simulink model "rah"  (Simulink 3.00)
settings: Solver=ode15s  SolverMode=SingleTasking  StartTime=0.0  StopTime=60  MaxStep=5  RelTol=1e-6  AbsTol=1e-6
undefined symbols (not defined in the file): Aail, Arud, Bail, Brud, Cail, Crud, Dail, dar, drr, Drud, Ki_2, Kphi, Kr, uaero0, uprop0, xinco
libraries: fbuttons x1, fdclib10 x1
settings Model: SaveTime=off  SaveOutput=off  RTWTemplateMakefile=grt_vc.tmf  LastModifiedBy=Dutchroll

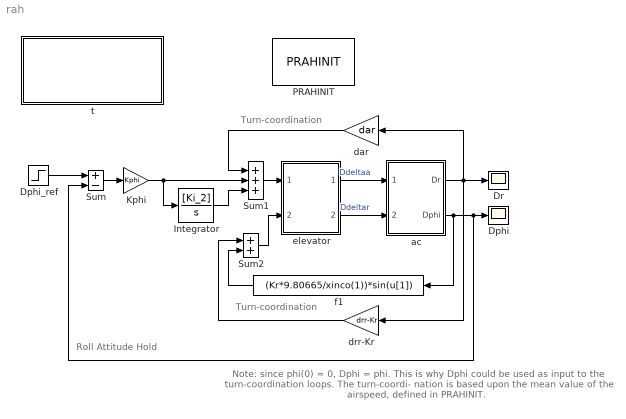
== system rah ==
  note: Note: since phi(0) = 0, Dphi = phi. This
      | is why Dphi could be used as input to the
      | turn-coordination loops. The turn-coordi-
      | nation is based upon the mean value of
      | the airspeed, defined in PRAHINIT.
  note: Roll Attitude Hold
  note: Turn-coordination
  note: Turn-coordination
  Dphi : Scope
      settings: TickLabels=on  TimeRange=60.000000  YMin=-0.3  YMax=0.3  SaveToWorkspace=off  SaveName=ScopeData  DataFormat=Matrix
  Dphi_ref : Step  Time=0  Before=0  After=10*pi/180  SampleTime=0
  Dr : Scope
      settings: TickLabels=on  TimeRange=60.000000  YMin=-0.025  YMax=0.025  SaveToWorkspace=off  SaveName=ScopeData  DataFormat=Matrix
  Integrator : TransferFcn  Numerator=[Ki_2]  Denominator=[1 0]
  Kphi : Gain  Gain=Kphi  SaturateOnIntegerOverflow=on
  PRAHINIT : fbuttons/PRAHINIT
  Sum : Sum  Inputs=+-  SaturateOnIntegerOverflow=on
  Sum1 : Sum  Inputs=+++  SaturateOnIntegerOverflow=on
  Sum2 : Sum  Inputs=++  SaturateOnIntegerOverflow=on
  ac : Subsystem
      mask Display: disp('BEAVER\ndynamics')
  dar : Gain  Orientation=left  Gain=dar  SaturateOnIntegerOverflow=on
  drr-Kr : Gain  Orientation=left  Gain=drr-Kr  SaturateOnIntegerOverflow=on
  elevator : Subsystem
      mask Display: disp('Cable &\nactuator\ndynamics')
  f1 : Fcn  Orientation=left  Expr=(Kr*9.80665/xinco(1))*sin(u[1])
  t : Subsystem
      settings: OpenFcn=browse apilot
      mask Display: disp('Roll Attitude Hold with\nturn-coordination\n(no signal limiters).\nM.O. Rauw, May 2004')
  wires:
  Dphi_ref/1 -> Sum/1
  Sum/1 -> Kphi/1
  elevator/1(Ddeltaa) -> ac/1(Ddelta_a)  "Ddeltaa"
  elevator/2(Ddeltar) -> ac/2(Ddelta_r)  "Ddeltar"
  Sum1/1 -> elevator/1(VDdeltaa)
  ac/1(Dr) -> Dr/1, dar/1, drr-Kr/1
  Sum2/1 -> elevator/2(VDdeltar)
  drr-Kr/1 -> Sum2/1
  ac/2(Dphi) -> Sum/2, Dphi/1, f1/1
  Kphi/1 -> Sum1/2, Integrator/1
  Integrator/1 -> Sum1/3
  dar/1 -> Sum1/1
  f1/1 -> Sum2/2

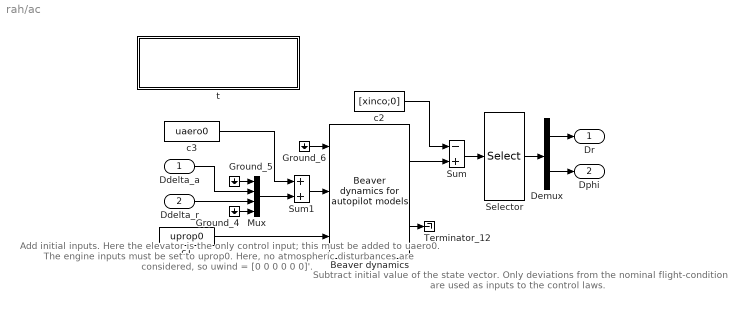
== system rah/ac ==
  note: Subtract initial value of  the state
      | vector. Only deviations from the
      | nominal flight-condition are used
      | as inputs to the control laws.
  note: Add initial inputs. Here the elevator
      | is the only control input; this must
      | be added to uaero0. The engine
      | inputs must be set to uprop0. Here,
      | no atmospheric disturbances are
      | considered, so uwind = [0 0 0 0 0 0]'.
  Ddelta_a : Inport  Port=1  PortWidth=-1  SampleTime=-1  DataType=auto
      settings: SignalType=auto
  Ddelta_r : Inport  Port=2  PortWidth=-1  SampleTime=-1  DataType=auto
      settings: SignalType=auto
  Beaver dynamics : fdclib10/Beaver dynamics for autopilot models
  Demux : Demux  Outputs=2
  Ground_4 : Ground
  Ground_5 : Ground
  Ground_6 : Ground
  Mux : Mux  Inputs=4
      settings: DisplayOption=none
  Selector : Selector  Elements=[6 9]  InputPortWidth=13
  Sum : Sum  Inputs=-+  SaturateOnIntegerOverflow=on
  Sum1 : Sum  Inputs=++  SaturateOnIntegerOverflow=on
  Terminator_12 : Terminator
  c1 : Constant  Value=uprop0
  c2 : Constant  Value=[xinco;0]
  c3 : Constant  Value=uaero0
  t : Subsystem
      mask Display: disp('Call aircraft model and convert\nI/O signals to small-deviations.\nM.O. Rauw, January 2004')
  Dr : Outport  Port=1
  Dphi : Outport  Port=2
  wires:
  c2/1 -> Sum/1
  Beaver dynamics/1 -> Sum/2
  Sum/1 -> Selector/1
  Beaver dynamics/2 -> Terminator_12/1
  Sum1/1 -> Beaver dynamics/2
  Ground_6/1 -> Beaver dynamics/1
  c3/1 -> Sum1/1
  Mux/1 -> Sum1/2
  Ddelta_a/1 -> Mux/2
  Ground_5/1 -> Mux/1
  Ddelta_r/1 -> Mux/3
  Ground_4/1 -> Mux/4
  c1/1 -> Beaver dynamics/3
  Selector/1 -> Demux/1
  Demux/1 -> Dr/1
  Demux/2 -> Dphi/1

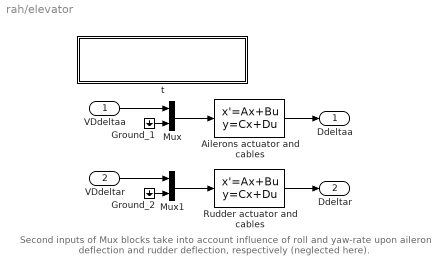
== system rah/elevator ==
  note: Second inputs of Mux blocks take into account
      | influence of roll and yaw-rate upon aileron deflection
      | and rudder deflection, respectively (neglected here).
  VDdeltaa : Inport  Port=1  PortWidth=-1  SampleTime=-1  DataType=auto
      settings: SignalType=auto
  VDdeltar : Inport  Port=2  PortWidth=-1  SampleTime=-1  DataType=auto
      settings: SignalType=auto
  Ailerons actuator and cables : StateSpace  A=Aail  B=Bail  C=Cail  D=Dail  X0=0
  Ground_1 : Ground
  Ground_2 : Ground
  Mux : Mux  Inputs=2
      settings: DisplayOption=none
  Mux1 : Mux  Inputs=2
      settings: DisplayOption=none
  Rudder actuator and cables : StateSpace  A=Arud  B=Brud  C=Crud  D=Drud  X0=0
  t : Subsystem
      settings: OpenFcn=browse actuatr
      mask Display: disp('Dynamics of the actuators and\ncables for ailerons and rudder.\nM.O. Rauw, April 2003')
  Ddeltaa : Outport  Port=1
  Ddeltar : Outport  Port=2
  wires:
  Ailerons actuator and cables/1 -> Ddeltaa/1
  VDdeltaa/1 -> Mux/1
  Mux/1 -> Ailerons actuator and cables/1
  Mux1/1 -> Rudder actuator and cables/1
  VDdeltar/1 -> Mux1/1
  Rudder actuator and cables/1 -> Ddeltar/1
  Ground_1/1 -> Mux/2
  Ground_2/1 -> Mux1/2

== system rah/t ==

== system rah/ac/t ==

== system rah/elevator/t ==
